simulink model "model_state_machine_Test"  (R2024a)
settings: Solver=VariableStepAuto  StartTime=0.0  StopTime=10.0  RelTol=1e-3
settings Model: Creator=Gabriel  LastModifiedBy=Gabriel

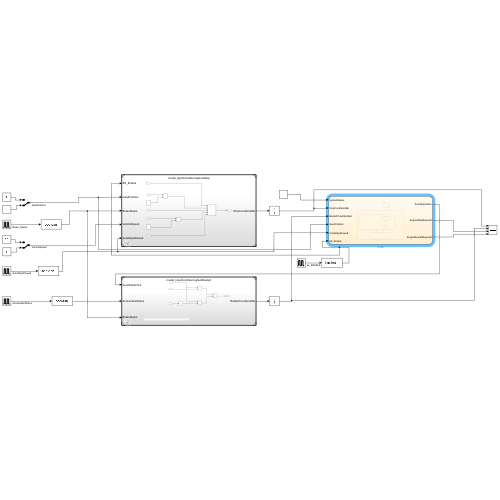
[thumbnail: Simulink's stored preview of the top-level diagram]
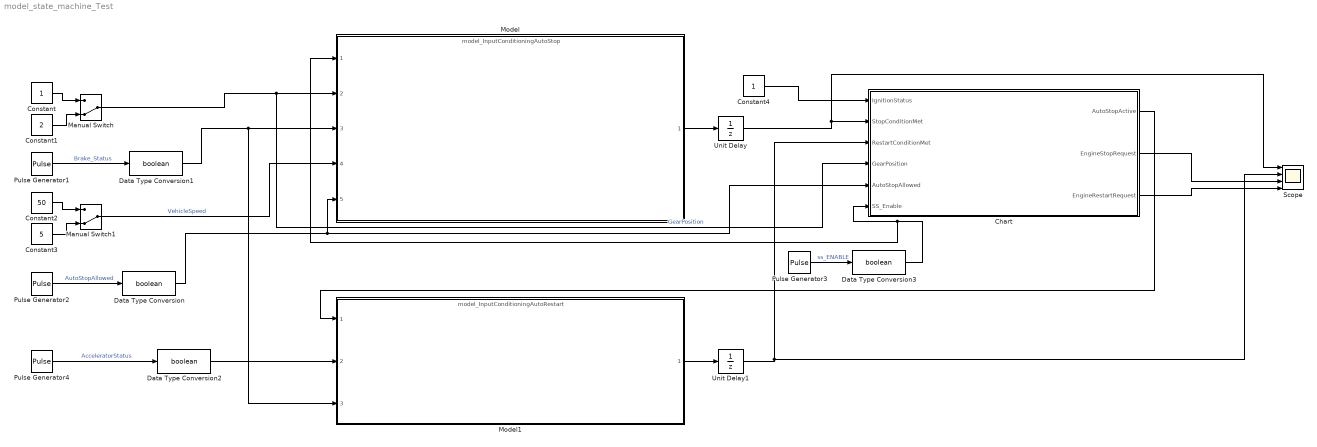
== system model_state_machine_Test ==
  Chart : Stateflow chart  TreatAsAtomicUnit=on
  Constant : Constant
  Constant1 : Constant  Value=2
  Constant2 : Constant  Value=50
  Constant3 : Constant  Value=5
  Constant4 : Constant  OutDataTypeStr=double
  Data Type Conversion{,1..3} (4 alike) : DataTypeConversion  OutDataTypeStr=boolean  SaturateOnIntegerOverflow=off  RndMeth=Floor
  Manual Switch : ManualSwitch  CurrentSetting=0
  Manual Switch1 : ManualSwitch  CurrentSetting=0
  Model : ModelReference  ModelNameDialog=model_InputConditioningAutoStop.slx  SimulationMode=Normal  ModelReferenceVersion=1.2
  Model1 : ModelReference  ModelNameDialog=model_InputConditioningAutoRestart.slx  SimulationMode=Normal  ModelReferenceVersion=1.3
  Pulse Generator1 : DiscretePulseGenerator  PulseType=Time based  PulseWidth=30
  Pulse Generator2 : DiscretePulseGenerator  PulseType=Time based  PulseWidth=60
  Pulse Generator3 : DiscretePulseGenerator  PulseType=Time based  Period=10  PulseWidth=50
  Pulse Generator4 : DiscretePulseGenerator  PulseType=Time based  PulseWidth=20
  Scope : Scope  NumInputPorts=4
  Unit Delay : UnitDelay  SampleTime=-1  HasFrameUpgradeWarning=on
  Unit Delay1 : UnitDelay  SampleTime=-1  HasFrameUpgradeWarning=on
  wires:
  Model/1 -> Unit Delay/1
  Pulse Generator1/1 -> Data Type Conversion1/1  "Brake_Status"
  Manual Switch1/1 -> Model/4  "VehicleSpeed"
  Constant2/1 -> Manual Switch1/1
  Constant/1 -> Manual Switch/1
  Pulse Generator2/1 -> Data Type Conversion/1  "AutoStopAllowed"
  Constant1/1 -> Manual Switch/2
  Constant3/1 -> Manual Switch1/2
  Manual Switch/1 -> Chart/4(GearPosition), Model/2  "GearPosition"
  Pulse Generator4/1 -> Data Type Conversion2/1  "AcceleratorStatus"
  Chart/1(AutoStopActive) -> Model1/1
  Chart/2(EngineStopRequest) -> Scope/3
  Chart/3(EngineRestartRequest) -> Scope/4
  Data Type Conversion/1 -> Chart/5(AutoStopAllowed), Model/5
  Data Type Conversion1/1 -> Model1/3, Model/3
  Data Type Conversion2/1 -> Model1/2
  Unit Delay/1 -> Chart/2(StopConditionMet), Scope/1
  Unit Delay1/1 -> Chart/3(RestartConditionMet), Scope/2
  Model1/1 -> Unit Delay1/1
  Constant4/1 -> Chart/1(IgnitionStatus)
  Pulse Generator3/1 -> Data Type Conversion3/1  "ss_ENABLE"
  Data Type Conversion3/1 -> Model/1, Chart/6(SS_Enable)

== stateflow chart model_state_machine_Test/Chart ==
  state VehicleOff
    entry:
    AutoStopActive =  false;
    EngineStopRequest = false;
    EngineRestartRequest =  false;
  state VehicleOn
    state SS_Available
      state EngineRunning
        entry:
        AutoStopActive = false;
        EngineStopRequest = false;
      state AutoStopActive
        entry:
        AutoStopActive = true;
        EngineRestartRequest = false;
      (default) -> EngineRunning
      AutoStopActive -> EngineRunning : [RestartConditionMet || GearPosition ~= 2 || after(180, sec)]{EngineRestartRequest = true;}
      EngineRunning -> AutoStopActive : [StopConditionMet]{EngineStopRequest = true;}
    state SS_Unavailable
      entry:
      AutoStopActive = false;
      EngineStopRequest = false;
      EngineRestartRequest = false;
    (default) -> SS_Available
    SS_Available -> SS_Unavailable : [SS_Enable == false]
    SS_Unavailable -> SS_Available : [SS_Enable == true]
  (default) -> VehicleOff
  VehicleOn -> VehicleOff : [IgnitionStatus ==  false]
  VehicleOff -> VehicleOn : [IgnitionStatus == true]
  data: IgnitionStatus input; StopConditionMet input; AutoStopActive output; RestartConditionMet input; EngineStopRequest output; EngineRestartRequest output; GearPosition input; AutoStopAllowed input; SS_Enable input
